simulink model "motorsim"  (R2023b)
settings: Solver=VariableStepAuto  StartTime=0.0  StopTime=50  RelTol=1e-3
values from neighbouring files (symbols this model uses):
  k = 1    [motor.m]
  k1 = 0.08    [motor.m]
  kE1 = 10    [motor.m]
  kE2 = 15    [motor.m]
  kem = 0.8    [motor.m]
  kEM = 0.02    [motor.m]
  kR = 5    [motor.m]
  T = 0.5    [motor.m]
  T1 = 0.05    [motor.m]
  Ti = 0.1    [motor.m]
  Tr = 1    [motor.m]
settings Model: Creator=Bianca  LastModifiedBy=Bianca

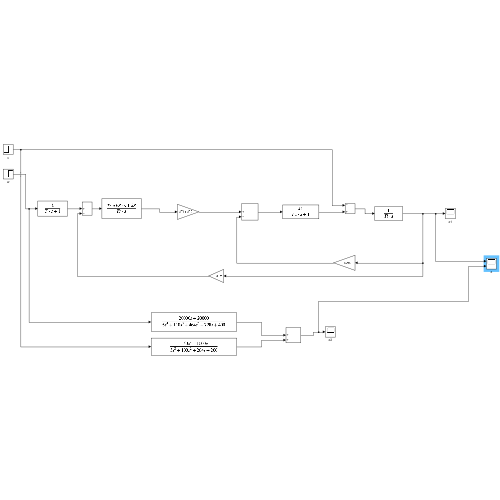
[thumbnail: Simulink's stored preview of the top-level diagram]
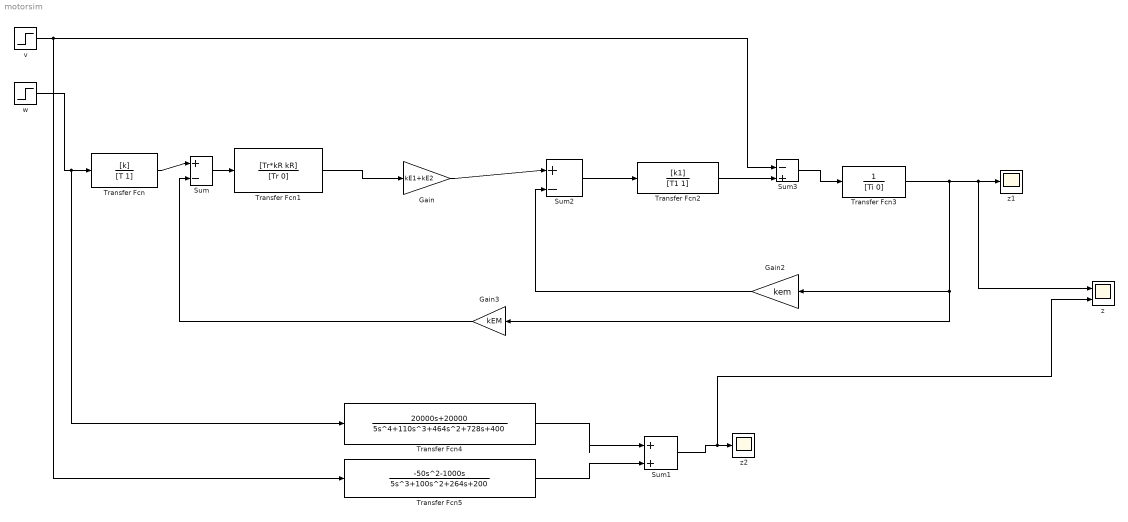
== system motorsim ==
  Gain : Gain  Gain=kE1+kE2
  Gain2 : Gain  Gain=kem
  Gain3 : Gain  Gain=kEM
  Sum : Sum  Inputs=|+-
  Sum1 : Sum  Inputs=|++
  Sum2 : Sum  Inputs=|+-
  Sum3 : Sum  Inputs=-|+
  Transfer Fcn : TransferFcn  Numerator=[k]  Denominator=[T 1]
  Transfer Fcn1 : TransferFcn  Numerator=[Tr*kR kR]  Denominator=[Tr 0]
  Transfer Fcn2 : TransferFcn  Numerator=[k1]  Denominator=[T1 1]
  Transfer Fcn3 : TransferFcn  Denominator=[Ti 0]
  Transfer Fcn4 : TransferFcn  Numerator=[20000 20000]  Denominator=[5 110 464 728 400]
  Transfer Fcn5 : TransferFcn  Numerator=[-50 -1000 0]  Denominator=[5 100 264 200]
  v : Step  Time=25  SampleTime=0
  w : Step  Time=0  After=5  SampleTime=0
  z : Scope  NumInputPorts=2
  z1 : Scope
  z2 : Scope
  wires:
  Transfer Fcn/1 -> Sum/1
  Sum/1 -> Transfer Fcn1/1
  Transfer Fcn1/1 -> Gain/1
  Gain/1 -> Sum2/1
  Sum2/1 -> Transfer Fcn2/1
  Transfer Fcn2/1 -> Sum3/2
  v/1 -> Transfer Fcn5/1, Sum3/1
  Sum3/1 -> Transfer Fcn3/1
  Transfer Fcn3/1 -> Gain3/1, Gain2/1, z/1, z1/1
  Gain2/1 -> Sum2/2
  w/1 -> Transfer Fcn4/1, Transfer Fcn/1
  Gain3/1 -> Sum/2
  Transfer Fcn4/1 -> Sum1/1
  Transfer Fcn5/1 -> Sum1/2
  Sum1/1 -> z/2, z2/1
